simulink model "pada_plant_model"  (R2022b)
settings: Solver=VariableStepAuto  StartTime=0.0  StopTime=1  RelTol=1e-3
values from neighbouring files (symbols this model uses):
  C_D0 = 0.0139    [pada_aero_coefficients.m]
  C_Dalpha = 0.2845    [pada_aero_coefficients.m]
  C_Dde = 0    [pada_aero_coefficients.m]
  C_Dq = 0    [pada_aero_coefficients.m]
  C_l0 = 0    [pada_aero_coefficients.m]
  C_L0 = 0.015    [pada_aero_coefficients.m]
  C_Lalpha = 2.60667    [pada_aero_coefficients.m]
  C_lbeta = -0.03987    [pada_aero_coefficients.m]
  C_lda = 0.21662    [pada_aero_coefficients.m]
  C_Lde = 0    [pada_aero_coefficients.m]
  C_Lq = 3.3277    [pada_aero_coefficients.m]
  C_m0 = 0.00035    [pada_aero_coefficients.m]
  C_malpha = -0.34517    [pada_aero_coefficients.m]
  C_mde = -0.44195    [pada_aero_coefficients.m]
  C_mq = -1.23417    [pada_aero_coefficients.m]
  C_n0 = 0    [pada_aero_coefficients.m]
  C_nbeta = 0.12715    [pada_aero_coefficients.m]
  C_nda = 0.00012    [pada_aero_coefficients.m]
  C_Xda = -0.00017    [pada_aero_coefficients.m]
  C_Xde = -0.00834    [pada_aero_coefficients.m]    (also in pada_linear_model.m = C_Xde)
  C_Y0 = 0    [pada_aero_coefficients.m]
  C_Ybeta = -0.63965    [pada_aero_coefficients.m]
  C_Yda = -0.02141    [pada_aero_coefficients.m]
  C_Yp = -0.06953    [pada_aero_coefficients.m]
  C_Yr = 0.51802    [pada_aero_coefficients.m]
  C_Zda = 0    [pada_aero_coefficients.m]
  C_Zde = -0.88788    [pada_aero_coefficients.m]    (also in pada_linear_model.m = C_Zde)
  g = 9.81    [pada_plant.m]
  J_x = 0.1    [pada_plant.m]
  J_xz = 0.0015    [pada_plant.m]
  J_y = 0.05    [pada_plant.m]
  J_z = 0.15    [pada_plant.m]
  k_motor = 20    [pada_plant.m]
  m = 0.4536    [pada_plant.m]
  Ref_area = 0.1039    [pada_plant.m]
  Ref_chord = 0.2472    [pada_plant.m]
  Ref_span = 0.4597    [pada_plant.m]
  rho = 1.225    [pada_plant.m]
  S_prop = 0.25    [pada_plant.m]
undefined symbols (not defined in the file or in its folder): K_lon
libraries: slpidlib x2, shared6dof x1, aerolibasang x1, sharedtransform x1, uavutilslib x1
settings Model: Creator=zachary  LastModifiedBy=zachary

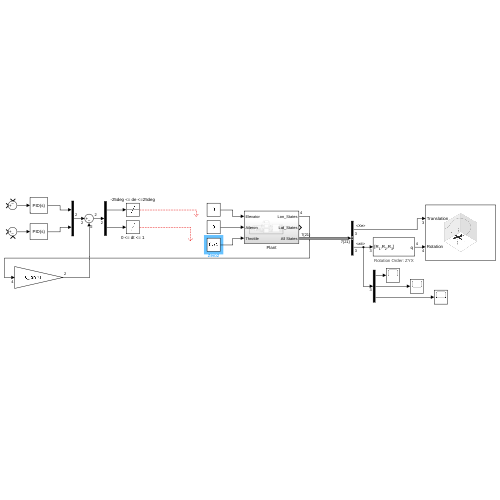
[thumbnail: Simulink's stored preview of the top-level diagram]
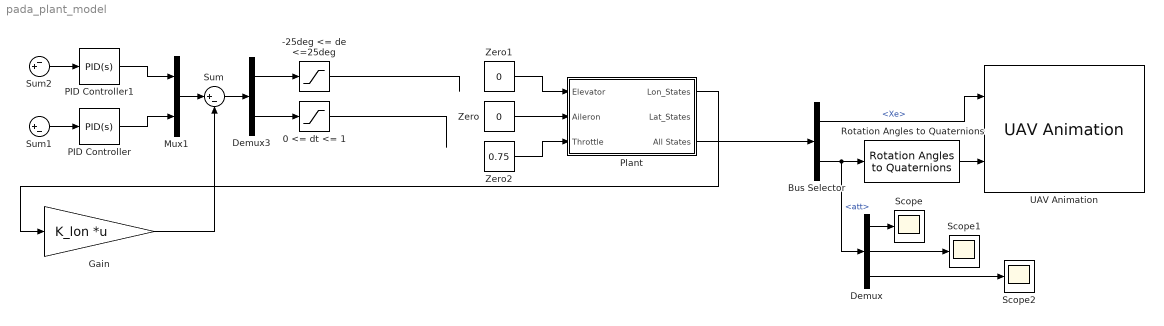
== system pada_plant_model ==
  -25deg <= de <=25deg : Saturate
  0 <= dt <= 1 : Saturate  UpperLimit=1  LowerLimit=0
  Bus Selector : BusSelector  OutputSignals=Xe,att
  Demux : Demux  Outputs=3
  Demux3 : Demux  Outputs=2
  Gain : Gain  Gain=K_lon  Multiplication=Matrix(K*u)
  Mux1 : Mux  Inputs=2
  PID Controller : slpidlib/PID Controller  Controller=PID  Form=Parallel  TimeDomain=Continuous-time  UseExternalTs=off  SampleTime=-1  IntegratorMethod=Forward Euler  FilterMethod=Forward Euler  ControllerParametersSource=internal  P=1  I=1  UseKiTs=off  D=0  N=100  UseFilter=on  TunerSelectOption=Transfer Function Based (PID Tuner App)  InitialConditionSource=internal  InitialConditionForIntegrator=0  InitialConditionForFilter=0  DifferentiatorICPrevScaledInput=0  ExternalReset=none  TrackingMode=off  Kt=1  LimitOutput=off  SatLimitsSource=internal  UpperSaturationLimit=inf  LowerSaturationLimit=-inf  LinearizeAsGain=on  AntiWindupMode=none  Kb=1  LimitIntegrator=off  UpperIntegratorSaturationLimit=inf  LowerIntegratorSaturationLimit=-inf  POutMin=[]  POutMax=[]  IOutMin=[]  IOutMax=[]  DOutMin=[]  DOutMax=[]  NOutMin=[]  NOutMax=[]  SumOutMin=[]  SumOutMax=[]  SaturationOutMin=[]  SaturationOutMax=[]  PParamMin=[]  PParamMax=[]  IParamMin=[]  IParamMax=[]  DParamMin=[]  DParamMax=[]  NParamMin=[]  NParamMax=[]  KbParamMin=[]  KbParamMax=[]  KtParamMin=[]  KtParamMax=[]  KbOutMin=[]  KbOutMax=[]  KtOutMin=[]  KtOutMax=[]  IntegratorOutMin=[]  IntegratorOutMax=[]  FilterOutMin=[]  FilterOutMax=[]  SumI1OutMin=[]  SumI1OutMax=[]  SumI2OutMin=[]  SumI2OutMax=[]  SumI3OutMin=[]  SumI3OutMax=[]  SumI4OutMin=[]  SumI4OutMax=[]  SumDOutMin=[]  SumDOutMax=[]  DifferentiatorOutMin=[]  DifferentiatorOutMax=[]  FilterDiffOutCoefMin=[]  FilterDiffOutCoefMax=[]  ReciprocalOutMin=[]  ReciprocalOutMax=[]  SumDenOutMin=[]  SumDenOutMax=[]  SumNumOutMin=[]  SumNumOutMax=[]  DivideOutMin=[]  DivideOutMax=[]  UdiffTsProdOutMin=[]  UdiffTsProdOutMax=[]  NTsProdOutMin=[]  NTsProdOutMax=[]  UintegralTsProdOutMin=[]  UintegralTsProdOutMax=[]  UngainTsProdOutMin=[]  UngainTsProdOutMax=[]  ClampingZeroOutDataTypeStr=Inherit: Inherit via back propagation  ClampingZeroOutMin=[]  ClampingZeroOutMax=[]  FilterDenConstantOutDataTypeStr=Inherit: Inherit via back propagation  FilterDenConstantOutMin=[]  FilterDenConstantOutMax=[]  PCopyOutDataTypeStr=Inherit: Inherit via back propagation  PCopyOutMin=[]  PCopyOutMax=[]  NCopyOutDataTypeStr=Inherit: Inherit via back propagation  NCopyOutMin=[]  NCopyOutMax=[]  IntegratorContinuousStateAttributes=''  IntegratorStateMustResolveToSignalObject=off  IntegratorRTWStateStorageClass=Auto  FilterContinuousStateAttributes=''  FilterStateMustResolveToSignalObject=off  FilterRTWStateStorageClass=Auto  ParallelPVariant=InternalParameters  IdealPVariant=Disabled  IVariant=InternalParameters  DVariant=InternalParameters  IntegratorVariant=Continuous  SatVariant=Disabled  AWVariant=Passthrough  PCopyVariant=Disabled  TRVariant=Disabled  FdbkBlocksVariant=Forward  IdealPFdbkVariant=Disabled  SatFdbkVariant=Disabled  DerivativeFilterVariant=ContFilter  NVariant=InternalParameters  NCopyVariant=Disabled  FilterICVariant=InternalICsFilter  IntegratorICVariant=InternalICs  ExternalResetVariant=Disabled  TRSumVariant=Passthrough  SumFdbkVariant=Disabled  SumVariant=Sum_PID  TsampFilterVariant=InternalTs  TsampNgainVariant=Passthrough  TsampIntegralVariant=Passthrough  ExternalSaturationOutDataTypeStr=Inherit: Same as second input
  PID Controller1 : slpidlib/PID Controller  Controller=PID  Form=Parallel  TimeDomain=Continuous-time  UseExternalTs=off  SampleTime=-1  IntegratorMethod=Forward Euler  FilterMethod=Forward Euler  ControllerParametersSource=internal  P=1  I=1  UseKiTs=off  D=0  N=100  UseFilter=on  TunerSelectOption=Transfer Function Based (PID Tuner App)  InitialConditionSource=internal  InitialConditionForIntegrator=0  InitialConditionForFilter=0  DifferentiatorICPrevScaledInput=0  ExternalReset=none  TrackingMode=off  Kt=1  LimitOutput=off  SatLimitsSource=internal  UpperSaturationLimit=inf  LowerSaturationLimit=-inf  LinearizeAsGain=on  AntiWindupMode=none  Kb=1  LimitIntegrator=off  UpperIntegratorSaturationLimit=inf  LowerIntegratorSaturationLimit=-inf  POutMin=[]  POutMax=[]  IOutMin=[]  IOutMax=[]  DOutMin=[]  DOutMax=[]  NOutMin=[]  NOutMax=[]  SumOutMin=[]  SumOutMax=[]  SaturationOutMin=[]  SaturationOutMax=[]  PParamMin=[]  PParamMax=[]  IParamMin=[]  IParamMax=[]  DParamMin=[]  DParamMax=[]  NParamMin=[]  NParamMax=[]  KbParamMin=[]  KbParamMax=[]  KtParamMin=[]  KtParamMax=[]  KbOutMin=[]  KbOutMax=[]  KtOutMin=[]  KtOutMax=[]  IntegratorOutMin=[]  IntegratorOutMax=[]  FilterOutMin=[]  FilterOutMax=[]  SumI1OutMin=[]  SumI1OutMax=[]  SumI2OutMin=[]  SumI2OutMax=[]  SumI3OutMin=[]  SumI3OutMax=[]  SumI4OutMin=[]  SumI4OutMax=[]  SumDOutMin=[]  SumDOutMax=[]  DifferentiatorOutMin=[]  DifferentiatorOutMax=[]  FilterDiffOutCoefMin=[]  FilterDiffOutCoefMax=[]  ReciprocalOutMin=[]  ReciprocalOutMax=[]  SumDenOutMin=[]  SumDenOutMax=[]  SumNumOutMin=[]  SumNumOutMax=[]  DivideOutMin=[]  DivideOutMax=[]  UdiffTsProdOutMin=[]  UdiffTsProdOutMax=[]  NTsProdOutMin=[]  NTsProdOutMax=[]  UintegralTsProdOutMin=[]  UintegralTsProdOutMax=[]  UngainTsProdOutMin=[]  UngainTsProdOutMax=[]  ClampingZeroOutDataTypeStr=Inherit: Inherit via back propagation  ClampingZeroOutMin=[]  ClampingZeroOutMax=[]  FilterDenConstantOutDataTypeStr=Inherit: Inherit via back propagation  FilterDenConstantOutMin=[]  FilterDenConstantOutMax=[]  PCopyOutDataTypeStr=Inherit: Inherit via back propagation  PCopyOutMin=[]  PCopyOutMax=[]  NCopyOutDataTypeStr=Inherit: Inherit via back propagation  NCopyOutMin=[]  NCopyOutMax=[]  IntegratorContinuousStateAttributes=''  IntegratorStateMustResolveToSignalObject=off  IntegratorRTWStateStorageClass=Auto  FilterContinuousStateAttributes=''  FilterStateMustResolveToSignalObject=off  FilterRTWStateStorageClass=Auto  ParallelPVariant=InternalParameters  IdealPVariant=Disabled  IVariant=InternalParameters  DVariant=InternalParameters  IntegratorVariant=Continuous  SatVariant=Disabled  AWVariant=Passthrough  PCopyVariant=Disabled  TRVariant=Disabled  FdbkBlocksVariant=Forward  IdealPFdbkVariant=Disabled  SatFdbkVariant=Disabled  DerivativeFilterVariant=ContFilter  NVariant=InternalParameters  NCopyVariant=Disabled  FilterICVariant=InternalICsFilter  IntegratorICVariant=InternalICs  ExternalResetVariant=Disabled  TRSumVariant=Passthrough  SumFdbkVariant=Disabled  SumVariant=Sum_PID  TsampFilterVariant=InternalTs  TsampNgainVariant=Passthrough  TsampIntegralVariant=Passthrough  ExternalSaturationOutDataTypeStr=Inherit: Same as second input
  Plant : Subsystem
  Rotation Angles to Quaternions : sharedtransform/Rotation Angles to Quaternions  rotationOrder=ZYX  aMode=aMode
  Scope : Scope
  Scope1 : Scope
  Scope2 : Scope
  Sum : Sum  Inputs=|+-
  Sum1 : Sum  Inputs=|+-
  Sum2 : Sum  Inputs=-+|
  UAV Animation : uavutilslib/UAV Animation  UAVType=FixedWing  UAVSize=1  InertialZDirection=Down  SampleTime=-1
  Zero : Constant  Value=0  OutDataTypeStr=Inherit: Inherit via back propagation
  Zero1 : Constant  Value=0  OutDataTypeStr=Inherit: Inherit via back propagation
  Zero2 : Constant  Value=0.75  OutDataTypeStr=Inherit: Inherit via back propagation
  wires:
  Demux3/1 -> -25deg <= de <=25deg/1
  Demux3/2 -> 0 <= dt <= 1/1
  Sum/1 -> Demux3/1
  Gain/1 -> Sum/2
  Mux1/1 -> Sum/1
  PID Controller/1 -> Mux1/2
  PID Controller1/1 -> Mux1/1
  Sum1/1 -> PID Controller/1
  Sum2/1 -> PID Controller1/1
  Plant/1(Lon_States) -> Gain/1
  -25deg <= de <=25deg/1 -> ?
  0 <= dt <= 1/1 -> ?
  Plant/3(All States) -> Bus Selector/1
  Bus Selector/1 -> UAV Animation/1  "<Xe>"
  Bus Selector/2 -> Demux/1, Rotation Angles to Quaternions/1  "<att>"
  Rotation Angles to Quaternions/1 -> UAV Animation/2
  Zero/1 -> Plant/2(Aileron)
  Zero2/1 -> Plant/3(Throttle)
  Zero1/1 -> Plant/1(Elevator)
  Demux/1 -> Scope/1
  Demux/2 -> Scope1/1
  Demux/3 -> Scope2/1

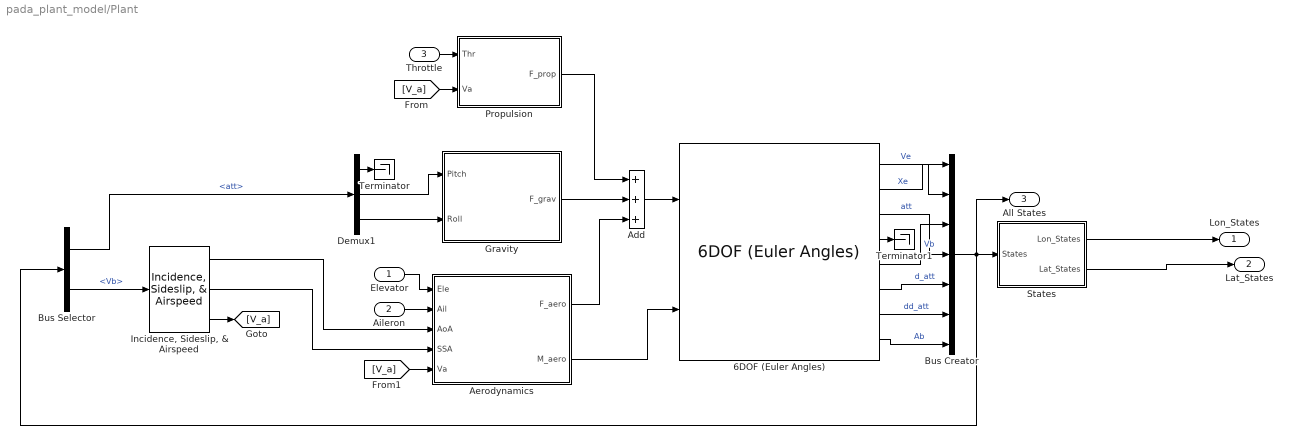
== system pada_plant_model/Plant ==
  Elevator : Inport
  Aileron : Inport  Port=2
  Throttle : Inport  Port=3
  6DOF (Euler Angles) : shared6dof/6DOF (Euler Angles)  units=Metric (MKS)  mtype=Fixed  rep=Euler Angles  xme_0=[0 0 0]  Vm_0=[0 0 0]  eul_0=[0 0 0]  pm_0=[0 0 0]  mass_0=m  mass_e=0.5  mass_f=2.0  inertia=[J_x, 0, -J_xz; 0, J_y, 0; -J_xz, 0, J_z]  inertia_e=eye(3)  inertia_f=2*eye(3)  k_quat=1.0  vre_flag=on  abi_flag=off  aMode=0  xme_statename=''  Vm_statename=''  eul_statename=''  quat_statename=''  pm_statename=''  mass_statename=''
  Add : Sum  Inputs=+++
  Aerodynamics : Subsystem
  Bus Creator : BusCreator  Inputs=7
  Bus Selector : BusSelector  OutputSignals=att,Vb
  Demux1 : Demux  Outputs=3
  Gravity : Subsystem
  "Incidence, Sideslip, & Airspeed" : aerolibasang/Incidence, Sideslip, & Airspeed
  Propulsion : Subsystem
  States : Subsystem
  Terminator : Terminator
  Terminator1 : Terminator
  Lon_States : Outport
  Lat_States : Outport  Port=2
  All States : Outport  Port=3
  wires:
  Bus Creator/1 -> All States/1, Bus Selector/1, States/1(States)
  Add/1 -> 6DOF (Euler Angles)/1
  Gravity/1(F_grav) -> Add/2
  Aerodynamics/1(F_aero) -> Add/3
  Propulsion/1(F_prop) -> Add/1
  "Incidence, Sideslip, & Airspeed"/2 -> Aerodynamics/4(SSA)
  Aerodynamics/2(M_aero) -> 6DOF (Euler Angles)/2
  "Incidence, Sideslip, & Airspeed"/1 -> Aerodynamics/3(AoA)
  Throttle/1 -> Propulsion/1(Thr)
  Elevator/1 -> Aerodynamics/1(Ele)
  6DOF (Euler Angles)/6 -> Bus Creator/5  "d_att"
  6DOF (Euler Angles)/4 -> Terminator1/1
  Aileron/1 -> Aerodynamics/2(Ail)
  Bus Selector/1 -> Demux1/1  "<att>"
  Demux1/1 -> Terminator/1
  6DOF (Euler Angles)/5 -> Bus Creator/3  "Vb"
  Demux1/2 -> Gravity/1(Pitch)
  6DOF (Euler Angles)/2 -> Bus Creator/1  "Xe"
  6DOF (Euler Angles)/7 -> Bus Creator/6  "dd_att"
  6DOF (Euler Angles)/8 -> Bus Creator/7  "Ab"
  6DOF (Euler Angles)/1 -> Bus Creator/2  "Ve"
  6DOF (Euler Angles)/3 -> Bus Creator/4  "att"
  Demux1/3 -> Gravity/2(Roll)
  Bus Selector/2 -> "Incidence, Sideslip, & Airspeed"/1  "<Vb>"
  States/2(Lat_States) -> Lat_States/1
  States/1(Lon_States) -> Lon_States/1
  [V_a] -> Propulsion/2(Va)
  [V_a] -> Aerodynamics/5(Va)
  "Incidence, Sideslip, & Airspeed"/3 -> [V_a]

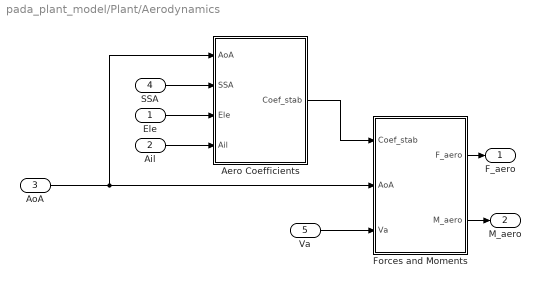
== system pada_plant_model/Plant/Aerodynamics ==
  Ele : Inport
  Ail : Inport  Port=2
  AoA : Inport  Port=3
  SSA : Inport  Port=4
  Va : Inport  Port=5
  Aero Coefficients : Subsystem
  Forces and Moments : Subsystem
  F_aero : Outport
  M_aero : Outport  Port=2
  wires:
  AoA/1 -> Forces and Moments/2(AoA), Aero Coefficients/1(AoA)
  Ail/1 -> Aero Coefficients/4(Ail)
  Forces and Moments/2(M_aero) -> M_aero/1
  Ele/1 -> Aero Coefficients/3(Ele)
  Aero Coefficients/1(Coef_stab) -> Forces and Moments/1(Coef_stab)
  Forces and Moments/1(F_aero) -> F_aero/1
  SSA/1 -> Aero Coefficients/2(SSA)
  Va/1 -> Forces and Moments/3(Va)

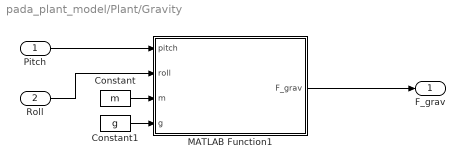
== system pada_plant_model/Plant/Gravity ==
  Pitch : Inport
  Roll : Inport  Port=2
  Constant : Constant  Value=m
  Constant1 : Constant  Value=g
  MATLAB Function1 : MATLAB Function  TreatAsAtomicUnit=on
  F_grav : Outport
  wires:
  Pitch/1 -> MATLAB Function1/1(pitch)
  MATLAB Function1/1(F_grav) -> F_grav/1
  Constant/1 -> MATLAB Function1/3(m)
  Constant1/1 -> MATLAB Function1/4(g)
  Roll/1 -> MATLAB Function1/2(roll)

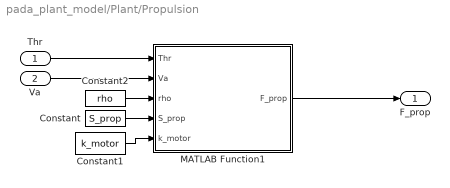
== system pada_plant_model/Plant/Propulsion ==
  Thr : Inport
  Va : Inport  Port=2
  Constant : Constant  Value=S_prop
  Constant1 : Constant  Value=k_motor
  Constant2 : Constant  Value=rho
  MATLAB Function1 : MATLAB Function  TreatAsAtomicUnit=on
  F_prop : Outport
  wires:
  MATLAB Function1/1(F_prop) -> F_prop/1
  Va/1 -> MATLAB Function1/2(Va)
  Constant2/1 -> MATLAB Function1/3(rho)
  Constant1/1 -> MATLAB Function1/5(k_motor)
  Constant/1 -> MATLAB Function1/4(S_prop)
  Thr/1 -> MATLAB Function1/1(Thr)

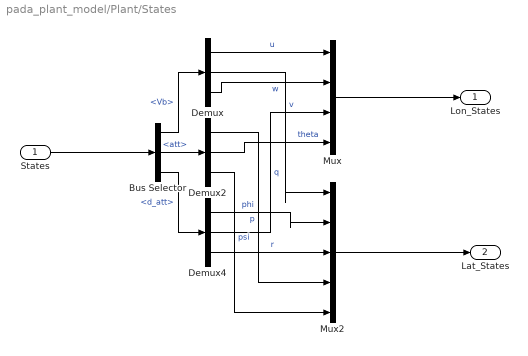
== system pada_plant_model/Plant/States ==
  States : Inport
  Bus Selector : BusSelector  OutputSignals=Vb,att,d_att
  Demux : Demux  Outputs=3
  Demux2 : Demux  Outputs=3
  Demux4 : Demux  Outputs=3
  Mux : Mux
  Mux2 : Mux  Inputs=5
  Lon_States : Outport
  Lat_States : Outport  Port=2
  wires:
  Demux/1 -> Mux/1  "u"
  Bus Selector/3 -> Demux4/1  "<d_att>"
  Demux/3 -> Mux/2  "w"
  Bus Selector/2 -> Demux2/1  "<att>"
  Demux4/2 -> Mux/3  "q"
  Demux2/1 -> Mux2/4  "phi"
  Bus Selector/1 -> Demux/1  "<Vb>"
  States/1 -> Bus Selector/1
  Demux/2 -> Mux2/1  "v"
  Demux4/3 -> Mux2/3  "r"
  Demux2/2 -> Mux/4  "theta"
  Demux4/1 -> Mux2/2  "p"
  Mux/1 -> Lon_States/1
  Mux2/1 -> Lat_States/1
  Demux2/3 -> Mux2/5  "psi"

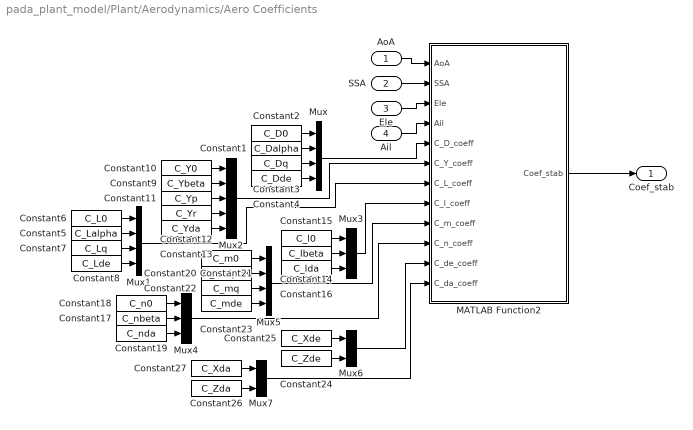
== system pada_plant_model/Plant/Aerodynamics/Aero Coefficients ==
  AoA : Inport
  SSA : Inport  Port=2
  Ele : Inport  Port=3
  Ail : Inport  Port=4
  Constant1 : Constant  Value=C_Dalpha
  Constant10 : Constant  Value=C_Y0
  Constant11 : Constant  Value=C_Yp
  Constant12 : Constant  Value=C_Yr
  Constant13 : Constant  Value=C_Yda
  Constant14 : Constant  Value=C_lbeta
  Constant15 : Constant  Value=C_l0
  Constant16 : Constant  Value=C_lda
  Constant17 : Constant  Value=C_nbeta
  Constant18 : Constant  Value=C_n0
  Constant19 : Constant  Value=C_nda
  Constant2 : Constant  Value=C_D0
  Constant20 : Constant  Value=C_malpha
  Constant21 : Constant  Value=C_m0
  Constant22 : Constant  Value=C_mq
  Constant23 : Constant  Value=C_mde
  Constant24 : Constant  Value=C_Zde
  Constant25 : Constant  Value=C_Xde
  Constant26 : Constant  Value=C_Zda
  Constant27 : Constant  Value=C_Xda
  Constant3 : Constant  Value=C_Dq
  Constant4 : Constant  Value=C_Dde
  Constant5 : Constant  Value=C_Lalpha
  Constant6 : Constant  Value=C_L0
  Constant7 : Constant  Value=C_Lq
  Constant8 : Constant  Value=C_Lde
  Constant9 : Constant  Value=C_Ybeta
  MATLAB Function2 : MATLAB Function  TreatAsAtomicUnit=on
  Mux : Mux
  Mux1 : Mux
  Mux2 : Mux  Inputs=5
  Mux3 : Mux  Inputs=3
  Mux4 : Mux  Inputs=3
  Mux5 : Mux
  Mux6 : Mux  Inputs=2
  Mux7 : Mux  Inputs=2
  Coef_stab : Outport
  wires:
  Constant23/1 -> Mux5/4
  Mux3/1 -> MATLAB Function2/8(C_l_coeff)
  Constant17/1 -> Mux4/2
  Constant14/1 -> Mux3/2
  Constant4/1 -> Mux/4
  Constant12/1 -> Mux2/4
  Mux2/1 -> MATLAB Function2/6(C_Y_coeff)
  Constant19/1 -> Mux4/3
  Constant18/1 -> Mux4/1
  Mux4/1 -> MATLAB Function2/10(C_n_coeff)
  Mux5/1 -> MATLAB Function2/9(C_m_coeff)
  Constant15/1 -> Mux3/1
  Constant16/1 -> Mux3/3
  SSA/1 -> MATLAB Function2/2(SSA)
  Constant7/1 -> Mux1/3
  Constant20/1 -> Mux5/2
  Constant5/1 -> Mux1/2
  Constant6/1 -> Mux1/1
  Constant8/1 -> Mux1/4
  Constant2/1 -> Mux/1
  MATLAB Function2/1(Coef_stab) -> Coef_stab/1
  Constant22/1 -> Mux5/3
  Constant9/1 -> Mux2/2
  Constant11/1 -> Mux2/3
  AoA/1 -> MATLAB Function2/1(AoA)
  Constant10/1 -> Mux2/1
  Mux/1 -> MATLAB Function2/5(C_D_coeff)
  Constant21/1 -> Mux5/1
  Constant3/1 -> Mux/3
  Constant13/1 -> Mux2/5
  Mux1/1 -> MATLAB Function2/7(C_L_coeff)
  Constant1/1 -> Mux/2
  Ele/1 -> MATLAB Function2/3(Ele)
  Ail/1 -> MATLAB Function2/4(Ail)
  Constant25/1 -> Mux6/1
  Constant24/1 -> Mux6/2
  Constant27/1 -> Mux7/1
  Constant26/1 -> Mux7/2
  Mux6/1 -> MATLAB Function2/11(C_de_coeff)
  Mux7/1 -> MATLAB Function2/12(C_da_coeff)

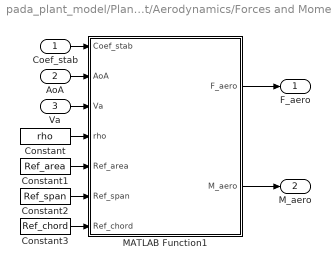
== system pada_plant_model/Plant/Aerodynamics/Forces and Moments ==
  Coef_stab : Inport
  AoA : Inport  Port=2
  Va : Inport  Port=3
  Constant : Constant  Value=rho
  Constant1 : Constant  Value=Ref_area
  Constant2 : Constant  Value=Ref_span
  Constant3 : Constant  Value=Ref_chord
  MATLAB Function1 : MATLAB Function  TreatAsAtomicUnit=on
  F_aero : Outport
  M_aero : Outport  Port=2
  wires:
  Constant3/1 -> MATLAB Function1/7(Ref_chord)
  Va/1 -> MATLAB Function1/3(Va)
  Constant1/1 -> MATLAB Function1/5(Ref_area)
  Constant/1 -> MATLAB Function1/4(rho)
  Coef_stab/1 -> MATLAB Function1/1(Coef_stab)
  AoA/1 -> MATLAB Function1/2(AoA)
  Constant2/1 -> MATLAB Function1/6(Ref_span)
  MATLAB Function1/1(F_aero) -> F_aero/1
  MATLAB Function1/2(M_aero) -> M_aero/1

== matlab function pada_plant_model/Plant/Aerodynamics/Forces and Moments/MATLAB Function1 ==
  data: Coef_stab input; AoA input; F_aero output size=[1 3]; M_aero output size=[1 3]; Va input; rho input; Ref_area input; Ref_span input; Ref_chord input
function [F_aero, M_aero]= AeroForcesInBody(Coef_stab, AoA, Va, rho, Ref_area, Ref_span, Ref_chord)

C_D = Coef_stab(1);
C_y = Coef_stab(2);
C_L = Coef_stab(3);
C_l = Coef_stab(4);
C_m = Coef_stab(5);
C_n = Coef_stab(6);

factor = 0.5 * rho * Va * Va * Ref_area;

F_lift = factor * C_L;
F_drag = factor * C_D;
F_x = -F_drag * cos(AoA) + F_lift * sin(AoA);
F_y = factor * C_y;
F_z = -F_drag * sin(AoA) - F_lift * cos(AoA);

l = factor * Ref_span * C_l;
m = factor * Ref_chord * C_m;
n = factor * Ref_span * C_n;

F_aero = [F_x, F_y, F_z];
M_aero = [l, m, n];

== matlab function pada_plant_model/Plant/Propulsion/MATLAB Function1 ==
  data: Thr input; F_prop output; Va input; rho input; S_prop input; k_motor input
function F_prop = ForcePropInBody(Thr, Va, rho, S_prop, k_motor)

F_xp = 0.5 * rho * S_prop * ((k_motor * Thr)^2 - Va);
F_prop = [F_xp, 0, 0];

== matlab function pada_plant_model/Plant/Aerodynamics/Aero Coefficients/MATLAB Function2 ==
  data: AoA input; SSA input; Coef_stab output; Ele input; Ail input; C_D_coeff input; C_Y_coeff input; C_L_coeff input; C_l_coeff input; C_m_coeff input; C_n_coeff input; C_de_coeff input; C_da_coeff input
function Coef_stab = AeroCoef(AoA, SSA, Ele, Ail, C_D_coeff, C_Y_coeff, C_L_coeff, C_l_coeff, C_m_coeff, C_n_coeff, C_de_coeff, C_da_coeff)

C_D0 = C_D_coeff(1);
C_Dalpha = C_D_coeff(2);
%C_Dq = C_D_coeff(3);
%C_Dde = C_D_coeff(4);

C_Y0 = C_Y_coeff(1);
C_Ybeta = C_Y_coeff(2);
%C_Yp = C_Y_coeff(3);
%C_Yr = C_Y_coeff(4);
C_Yda = C_Y_coeff(5);

C_L0 = C_L_coeff(1);
C_Lalpha = C_L_coeff(2);
%C_Lq = C_L_coeff(3);
%C_Lde = C_L_coeff(4);

C_l0 = C_l_coeff(1);
C_lbeta = C_l_coeff(2);
C_lda = C_l_coeff(3);

C_m0 = C_m_coeff(1);
C_malpha = C_m_coeff(2);
%C_mq = C_m_coeff(3);
C_mde = C_m_coeff(4);

C_n0 = C_n_coeff(1);
C_nbeta = C_n_coeff(2);
C_nda = C_n_coeff(3);

C_Xde = C_de_coeff(1);
C_Zde = C_de_coeff(2);

%C_Xda = C_da_coeff(1);
%C_Zda = C_da_coeff(2);

C_Dde = -C_Xde*cos(AoA) - C_Zde*sin(AoA);
C_Lde = C_Xde*sin(AoA) - C_Zde*cos(AoA);

% F_x = -F_drag * cos(AoA) + F_lift * sin(AoA);
% F_y = factor * C_y;
% F_z = -F_drag * sin(AoA) - F_lift * cos(AoA);

C_D = C_D0 + C_Dalpha * AoA + C_Dde * Ele;
C_Y = C_Y0 + C_Ybeta * SSA + C_Yda * Ail;
C_L = C_L0 + C_Lalpha * AoA + C_Lde * Ele;
C_l = C_l0 + C_lbeta * SSA + C_lda * Ail;
C_m = C_m0 + C_malpha * AoA + C_mde * Ele;
C_n = C_n0 + C_nbeta * SSA + C_nda * Ail;

Coef_stab = [C_D, C_Y, C_L, C_l, C_m, C_n];

== matlab function pada_plant_model/Plant/Gravity/MATLAB Function1 ==
  data: pitch input; F_grav output; roll input; m input; g input
function F_grav = GravityInBody(pitch, roll, m, g)

F_gx = -m*g*sin(pitch);
F_gy = m*g*cos(pitch)*sin(roll);
F_gz = m*g*cos(pitch)*cos(roll);

F_grav = [F_gx, F_gy, F_gz];
